simulink model "dspchanest"  (Simulink 8.3)
settings: Solver=FixedStepDiscrete  StartTime=0.0  StopTime=999999  RelTol=1e-3
undefined symbols (not defined in the file or in its folder): dfilt
libraries: simulink x3, dsparch4 x2, dspmisc x1, dspmtrx3 x1, dspadpt3 x1
settings Model: Creator=The MathWorks Inc.  ExtModeAutoUpdateStatusClock=off
settings SolverCC: InsertRTBMode=Auto
settings OptimizationCC: ExpressionDepthLimit=2147483647  InitFltsAndDblsToZero=on
settings DebuggingCC: FcnCallInpInsideContextMsg=UseLocalSettings  StrictBusMsg=Warning

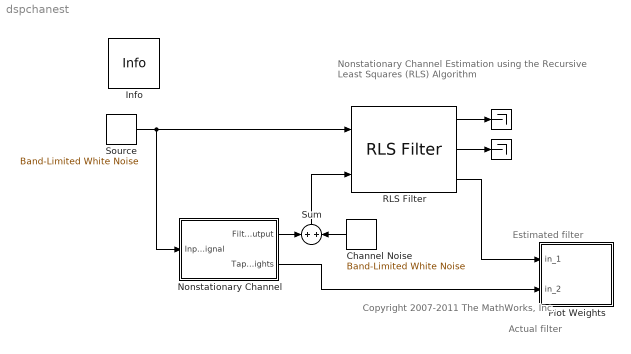
== system dspchanest ==
  note: Nonstationary Channel Estimation
      | using the Recursive Least Squares (RLS) Algorithm
  note: Estimated
      | filter
  note: Actual
      | filter
  note: Copyright 2007-2011 The MathWorks, Inc.
  " " : Terminator
  "  " : Terminator
  Channel Noise : simulink/Sources/Band-Limited White Noise  Cov=.3  Ts=1  seed=12345
  Info : dspmisc/Info  SystemSampleTime=-1
  Nonstationary Channel : Subsystem  mask{N=5, a=0.96, Ts=1}
      mask prompts: N "Filter Order:"; a "Nonstationarity Parameter (0 to 1):"; Ts "Sample Time:"
      mask help: Nonstationary Nth Order Noisy Channel
      mask Help: Implementation of a nonstationary filter.  Nonstationarity parameter controls the filter tap nonstationarity, and may take values in the range 0 <= a < 1.  The first system output is the actual filter taps over time, and the second output is a vector of instantaneous tap weight estimates ("unknowns")
      mask Display: disp('Nonstationary\nSystem')
  Plot Weights : Subsystem
      mask Display: disp('Plot\nWeights')
  RLS Filter : dspadpt3/RLS Filter  L=5  lambdaflag=Dialog  lambda=.85  addnparflag=on  ic=0  delta=0.1  Adapt=off  resetflag=None  weights=on
  Source : simulink/Sources/Band-Limited White Noise  Cov=[0.1]  Ts=1  seed=[23341]
  Sum : Sum  Inputs=+|+  SaturateOnIntegerOverflow=on  InputSameDT=on  OutDataTypeStr=Inherit: Same as first input
  wires:
  Source/1 -> RLS Filter/1, Nonstationary Channel/1(Input Signal)
  Channel Noise/1 -> Sum/2
  Sum/1 -> RLS Filter/2
  RLS Filter/1 -> " "/1
  RLS Filter/2 -> "  "/1
  Nonstationary Channel/2(Tap Weights) -> Plot Weights/2(in_2)
  Nonstationary Channel/1(Filter Output) -> Sum/1
  RLS Filter/3 -> Plot Weights/1(in_1)

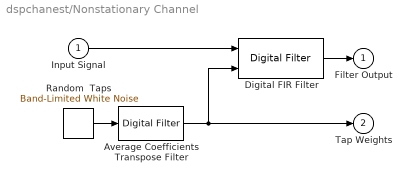
== system dspchanest/Nonstationary Channel ==
  Input Signal : Inport
  Average Coefficients Transpose Filter : dsparch4/Digital Filter  TypePopup=IIR (all poles)  IIRFiltStruct=Direct form II transposed  AllPoleFiltStruct=Direct form transposed  FIRFiltStruct=Direct form  CoeffSource=Specify via dialog  NumCoeffs=[1 2]  DenCoeffs=[1 -a]  BiQuadCoeffs=[1 0.3 0.4 1 0.1 0.2]  LatticeCoeffs=[0.2 0.4]  denIgnore=on  FiltPerSampPopup=One filter per frame  IC=0  ICnum=0  ICden=0  roundingMode=Floor  overflowMode=off  ScaleValues=1  scaleValueFracLength=14  stageInFracLength=15  stageOutFracLength=15  FilterSource=Specify via dialog  dfiltObjectName=dfilt.dffir([1 2 1])
  Digital FIR Filter : dsparch4/Digital Filter  TypePopup=FIR (all zeros)  IIRFiltStruct=Direct form II transposed  AllPoleFiltStruct=Direct form  FIRFiltStruct=Direct form transposed  CoeffSource=Input port(s)  NumCoeffs=[1 2]  DenCoeffs=[1 0.1]  BiQuadCoeffs=[1 0.3 0.4 1 0.1 0.2]  LatticeCoeffs=[0.2 0.4]  denIgnore=on  FiltPerSampPopup=One filter per sample  IC=0  ICnum=0  ICden=0  roundingMode=Floor  overflowMode=off  ScaleValues=1  scaleValueFracLength=14  stageInFracLength=15  stageOutFracLength=15  FilterSource=Input port(s)  dfiltObjectName=dfilt.dffir([1 2 1])
  Random  Taps : simulink/Sources/Band-Limited White Noise  Cov=ones(N,1)  Ts=Ts  seed=round(rand(N,1)*1000)
  Filter Output : Outport
  Tap Weights : Outport  Port=2
  wires:
  Input Signal/1 -> Digital FIR Filter/1
  Digital FIR Filter/1 -> Filter Output/1
  Random  Taps/1 -> Average Coefficients Transpose Filter/1
  Average Coefficients Transpose Filter/1 -> Tap Weights/1, Digital FIR Filter/2

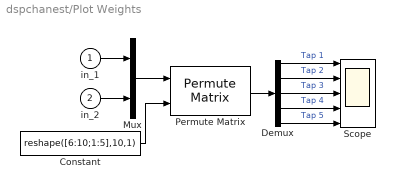
== system dspchanest/Plot Weights ==
  in_1 : Inport
  in_2 : Inport  Port=2
  Constant : Constant  Value=reshape([6:10;1:5],10,1)
  Demux : Demux  Outputs=5
  Mux : Mux  Inputs=2
  Permute Matrix : dspmtrx3/Permute Matrix  mode=Rows  ZeroOneIdxMode=One-based  errmode=Clip index  checkDims=off
  Scope : Scope  NumInputPorts=5
      settings: TimeRange=300  YMin=-10~-10~-10~-10~-10  YMax=10~10~10~10~10  DataFormat=Structure  SampleInput=on
  wires:
  Demux/5 -> Scope/5  "Tap 5"
  in_1/1 -> Mux/1
  in_2/1 -> Mux/2
  Mux/1 -> Permute Matrix/1
  Constant/1 -> Permute Matrix/2
  Permute Matrix/1 -> Demux/1
  Demux/1 -> Scope/1  "Tap 1"
  Demux/4 -> Scope/4  "Tap 4"
  Demux/3 -> Scope/3  "Tap 3"
  Demux/2 -> Scope/2  "Tap 2"
